simulink model "OFDM"  (R2021a)
settings: Solver=VariableStepAuto  StartTime=0.0  StopTime=20  RelTol=1e-3
undefined symbols (not defined in the file): M, N, nbPilots, nbZeros, nCycle, nTotal, nUtile, Ts
libraries: dspxfrm3 x2, commdigbbndpm3 x2, commchan3 x1, commrandsrc3 x1
settings Model: Creator=PC  LastModifiedBy=ayoub
settings SolverCC: AlgebraicLoopSolver=TrustRegion
settings DebuggingCC: UnconnectedInputMsg=none  UnconnectedOutputMsg=none  UnconnectedLineMsg=none
settings ModelReferenceCC: EnableRefExpFcnMdlSchedulingChecks=off
settings SFSimCC: CustomCodeUndefinedFunction=UseInterfaceOnly
settings RTWCC: Description=Generic Real-Time Target

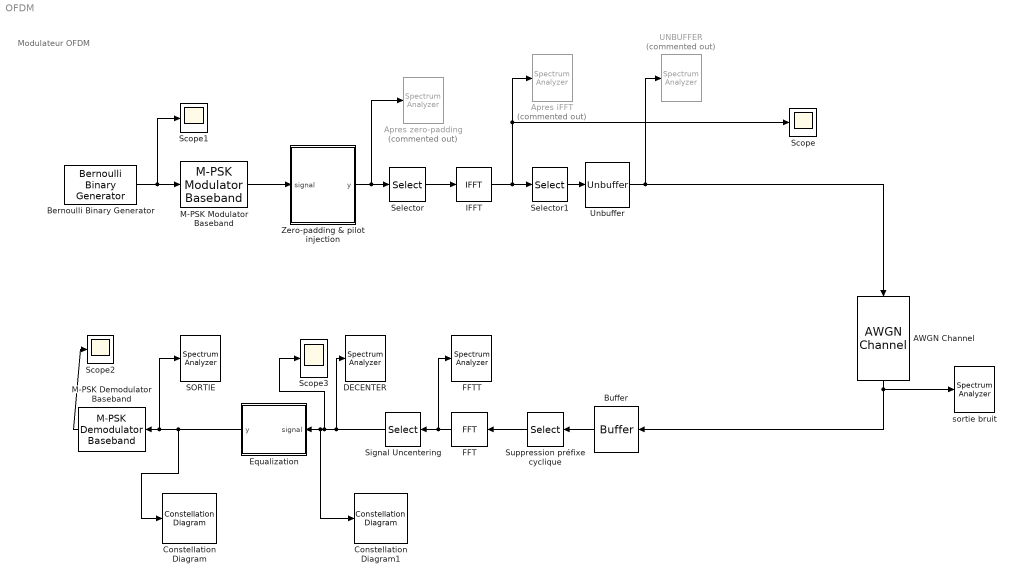
== system OFDM ==
  note: Modulateur OFDM
  AWGN Channel : commchan3/AWGN Channel  InputProcessing=Columns as channels (frame based)  seed=67  noiseMode="Signal to noise ratio  (SNR)"  EbNodB=10  EsNodB=10  SNRdB=SNR_  bitsPerSym=1  Ps=1  Tsym=1  variance=1
  Apres iFFT : SpectrumAnalyzer  Commented=on
  Apres zero-padding : SpectrumAnalyzer  Commented=on
  Bernoulli Binary Generator : commrandsrc3/Bernoulli Binary Generator  ProbabilityOfZero=0.5  SeedSource=Auto  Seed=0  SampleTime=Ts/(nUtile*M)  SamplesPerFrame=nUtile*M  OutputDataType=double  SimulateUsing=Code generation
  Buffer : Buffer  N=nTotal  OutputFrames=off
  Constellation Diagram : ConstellationDiagram
  Constellation Diagram1 : ConstellationDiagram
  DECENTER : SpectrumAnalyzer
  Equalization : MATLAB Function  TreatAsAtomicUnit=on
  FFT : dspxfrm3/FFT  FFTImplementation=Auto  CompMethod=Table lookup  TableOpt=NEW  TableOptActive=Speed  BitRevOrder=off  Normalize=off  InheritFFTLength=on  FFTLength=64  WrapInput=on  roundingMode=Floor  overflowMode=off  firstCoeffDataTypeStr=Inherit: Same word length as input  firstCoeffLastDataTypeStr=Inherit: Same word length as input  outputMin=[]  outputMax=[]
  FFTT : SpectrumAnalyzer
  IFFT : dspxfrm3/IFFT  FFTImplementation=Auto  CompMethod=Table lookup  TableOpt=NEW  TableOptActive=Speed  BitRevOrder=off  cs_in=off  Normalize=on  InheritFFTLength=on  FFTLength=64  WrapInput=on  mode=Complex  outSamplingMode=Sample based  roundingMode=Floor  overflowMode=off  firstCoeffDataTypeStr=Inherit: Same word length as input  firstCoeffLastDataTypeStr=Inherit: Same word length as input  outputMin=[]  outputMax=[]
  M-PSK Demodulator Baseband : commdigbbndpm3/M-PSK Demodulator Baseband  M=8  OutType=Integer  DecType=Hard decision  VarSource=Dialog  Variance=1  Dec=Gray  Mapping=[0:7]  Ph=pi/8  outDtype1=Inherit via internal rule  outDtype2=Inherit via internal rule  derotateFactorWordLen=16  derotateFactorDataTypeStr=Inherit: Same word length as input  derotateFactorLastDataTypeStr=Inherit: Same word length as input
  M-PSK Modulator Baseband : commdigbbndpm3/M-PSK Modulator Baseband  M=2^M  InType=Bit  Enc=Gray  Mapping=[0:7]  Ph=pi/(2^M)  outDtype=double  outWordLen=16  outUDDataType=sfix(16)  outFracLenMode=Best precision  outFracLen=15  outDataTypeStr=double  outLastDataTypeStr=double
  SORTIE : SpectrumAnalyzer
  Scope{,1..3} (4 alike) : Scope
  Selector : Selector  InputPortWidth=N  IndexOptions=Index vector (dialog)  Indices=[N/2:N 1:N/2-1]  OutputSizes=1
  Selector1 : Selector  InputPortWidth=N  IndexOptions=Index vector (dialog)  Indices=[N-nCycle + 1:N 1:N]  OutputSizes=1
  Signal Uncentering : Selector  InputPortWidth=N  IndexOptions=Index vector (dialog)  Indices=[N/2+2:N 1:N/2+1]  OutputSizes=1
  Suppression préfixe cyclique : Selector  InputPortWidth=nTotal  IndexOptions=Index vector (dialog)  Indices=[nCycle+1:nTotal]  OutputSizes=1
  UNBUFFER : SpectrumAnalyzer  Commented=on
  Unbuffer : Unbuffer
  Zero-padding & pilot injection : MATLAB Function  TreatAsAtomicUnit=on
  sortie bruit : SpectrumAnalyzer
  wires:
  Bernoulli Binary Generator/1 -> Scope1/1, M-PSK Modulator Baseband/1
  M-PSK Modulator Baseband/1 -> Zero-padding & pilot injection/1(signal)
  Zero-padding & pilot injection/1(y) -> Selector/1, Apres zero-padding/1
  Selector/1 -> IFFT/1
  IFFT/1 -> Selector1/1, Scope/1, Apres iFFT/1
  Unbuffer/1 -> AWGN Channel/1, UNBUFFER/1
  Selector1/1 -> Unbuffer/1
  Suppression préfixe cyclique/1 -> FFT/1
  Signal Uncentering/1 -> DECENTER/1, Scope3/1, Constellation Diagram1/1, Equalization/1(signal)
  Buffer/1 -> Suppression préfixe cyclique/1
  FFT/1 -> FFTT/1, Signal Uncentering/1
  AWGN Channel/1 -> Buffer/1, sortie bruit/1
  Equalization/1(y) -> Constellation Diagram/1, SORTIE/1, M-PSK Demodulator Baseband/1
  M-PSK Demodulator Baseband/1 -> Scope2/1

== matlab function OFDM/Equalization ==
  data: y output size=[nUtile,1]; signal input; nbPilots parameter; nUtile parameter; nbZeros parameter
function y = fcn(signal, nbPilots, nUtile, nbZeros)

    signalSansZeros = signal(nbZeros/2+1:nbZeros/2+nUtile+nbPilots);

    intervalle = floor(nUtile/nbPilots)+1;
    output = zeros(nUtile,1) + 1j * zeros(nUtile,1);
    indexOutput = 1;
    
    coeffs = zeros(nbPilots,1)+ 1j*zeros(nbPilots,1);
    indexCoeffs = 1;
    indexes = zeros(nbPilots,1);
    indexIndexes = 1;
    
    for i = 1:nUtile+nbPilots
        if mod(i+floor(intervalle/2),intervalle) == 0
            if (indexCoeffs <= nbPilots)
                coeffs(indexCoeffs) = (sqrt(2)+sqrt(2)*1j)/signalSansZeros(i);
                indexes(indexIndexes) = i;
                indexCoeffs = indexCoeffs + 1;
                indexIndexes = indexIndexes + 1;
            end
        end
    end
    
    coeffsInterp = interp1(indexes,coeffs,1:nUtile+nbPilots,'spline');
    
    coeffsInterp(1:intervalle) = coeffs(1);
    coeffsInterp(nUtile+nbPilots-intervalle:end) = coeffs(nbPilots);
    
    for i = 1:nUtile+nbPilots
        if mod(i+floor(intervalle/2),intervalle) ~= 0
            output(indexOutput) = signalSansZeros(i)*coeffsInterp(i);
            indexOutput = indexOutput + 1;
        end
    end

y = output;

== matlab function OFDM/Zero-padding & pilot injection ==
  data: y output size=[N,1]; nbZeros parameter; nbPilots parameter; signal input size=nUtile; nUtile parameter
function y = fcn(nbZeros, nbPilots, signal, nUtile)

    index = 1;
    
    intervalle = floor(nUtile/nbPilots)+1;
    output = zeros(nbZeros+nbPilots+nUtile,1)+1j * zeros(nbZeros+nbPilots+nUtile,1);
    
    for i=nbZeros/2+1:nUtile+nbZeros/2+nbPilots
        if mod(i-nbZeros/2+floor(intervalle/2),intervalle) == 0
            output(i)= sqrt(2)+sqrt(2)*1j;
        else
            output(i)=signal(index);
            index = index+1;
        end
    end
y = output;
